simulink model "integrator_test"  (R2021b)
settings: Solver=FixedStepAuto  StartTime=0.0  StopTime=30e-4  FixedStep=4e-9  RelTol=1e-3
values from neighbouring files (symbols this model uses):
  force_func = @(x) p.alpha * x.^3 - p.beta * x    [hilsim_playground.m]
undefined symbols (not defined in the file or in its folder): hw, m, p, renorm_x
settings Model: Creator=berndorfer  LastModifiedBy=berndorfer

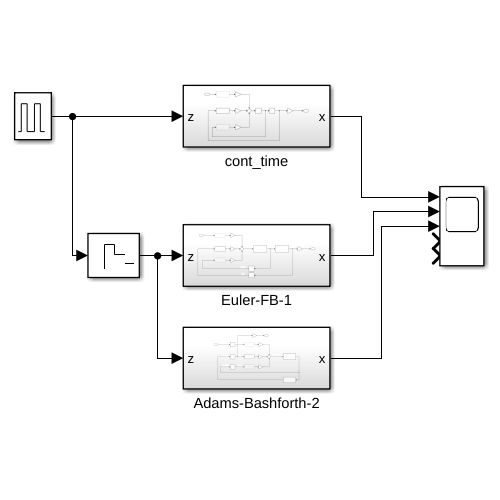
[thumbnail: Simulink's stored preview of the top-level diagram]
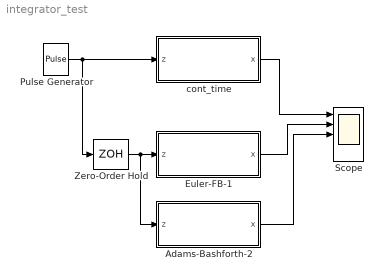
== system integrator_test ==
  Adams-Bashforth-2 : Subsystem
  Euler-FB-1 : Subsystem
  Pulse Generator : DiscretePulseGenerator  PulseType=Time based  Amplitude=-1  Period=2e-3  PulseWidth=4  PhaseDelay=0.05e-3
  Scope : Scope  NumInputPorts=5
  Zero-Order Hold : ZeroOrderHold  SampleTime=hw.t_s * hw.oversample
  cont_time : Subsystem
  wires:
  Pulse Generator/1 -> Zero-Order Hold/1, cont_time/1(z)
  cont_time/1(x) -> Scope/1
  Euler-FB-1/1(x) -> Scope/2
  Adams-Bashforth-2/1(x) -> Scope/3
  Zero-Order Hold/1 -> Adams-Bashforth-2/1(z), Euler-FB-1/1(z)

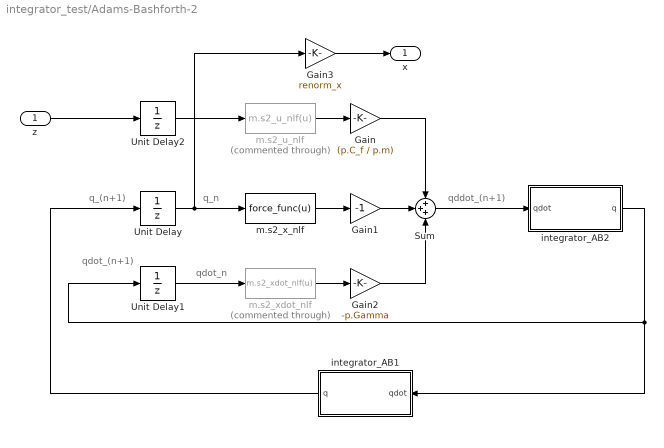
== system integrator_test/Adams-Bashforth-2 ==
  note: q_n
  note: qddot_(n+1)
  note: qdot_(n+1)
  note: qdot_n
  note: q_(n+1)
  z : Inport
  Gain : Gain  Gain=(p.C_f / p.m)
  Gain1 : Gain  Gain=-1
  Gain2 : Gain  Gain=-p.Gamma
  Gain3 : Gain  Gain=renorm_x
  Sum : Sum  Inputs=+++
  Unit Delay : UnitDelay  SampleTime=hw.t_s * hw.oversample  HasFrameUpgradeWarning=on
  Unit Delay1 : UnitDelay  SampleTime=hw.t_s * hw.oversample  HasFrameUpgradeWarning=on
  Unit Delay2 : UnitDelay  SampleTime=hw.t_s * hw.oversample  HasFrameUpgradeWarning=on
  integrator_AB1 : Subsystem
  integrator_AB2 : Subsystem
  m.s2_u_nlf : MATLABFcn  Commented=through  MATLABFcn=m.s2_u_nlf(u)  OutputDimensions=1
  m.s2_x_nlf : MATLABFcn  MATLABFcn=force_func(u)  OutputDimensions=1
  m.s2_xdot_nlf : MATLABFcn  Commented=through  MATLABFcn=m.s2_xdot_nlf(u)  OutputDimensions=1
  x : Outport
  wires:
  Gain1/1 -> Sum/2
  z/1 -> Unit Delay2/1
  Gain/1 -> Sum/1
  m.s2_x_nlf/1 -> Gain1/1
  Unit Delay/1 -> Gain3/1, m.s2_x_nlf/1
  m.s2_xdot_nlf/1 -> Gain2/1
  Gain2/1 -> Sum/3
  m.s2_u_nlf/1 -> Gain/1
  Gain3/1 -> x/1
  Unit Delay2/1 -> m.s2_u_nlf/1
  Unit Delay1/1 -> m.s2_xdot_nlf/1
  integrator_AB2/1(q) -> integrator_AB1/1(qdot), Unit Delay1/1
  integrator_AB1/1(q) -> Unit Delay/1
  Sum/1 -> integrator_AB2/1(qdot)

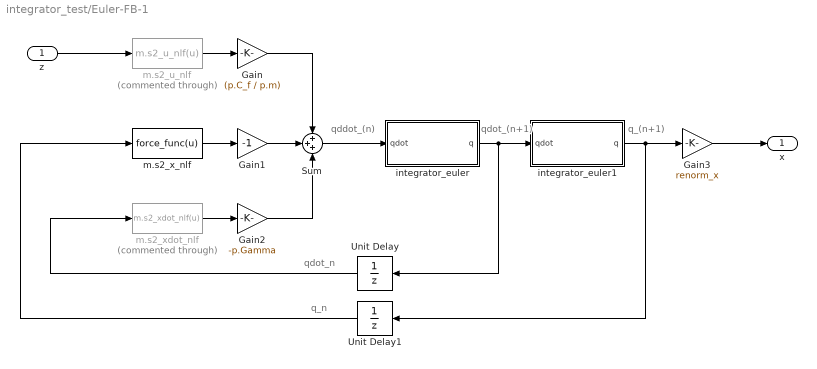
== system integrator_test/Euler-FB-1 ==
  note: qdot_n
  note: qdot_(n+1)
  note: q_(n+1)
  note: q_n
  note: qddot_(n)
  z : Inport
  Gain : Gain  Gain=(p.C_f / p.m)
  Gain1 : Gain  Gain=-1
  Gain2 : Gain  Gain=-p.Gamma
  Gain3 : Gain  Gain=renorm_x
  Sum : Sum  Inputs=+++
  Unit Delay : UnitDelay  SampleTime=hw.t_s * hw.oversample  HasFrameUpgradeWarning=on
  Unit Delay1 : UnitDelay  SampleTime=hw.t_s * hw.oversample  HasFrameUpgradeWarning=on
  integrator_euler : Subsystem
  integrator_euler1 : Subsystem
  m.s2_u_nlf : MATLABFcn  Commented=through  MATLABFcn=m.s2_u_nlf(u)  OutputDimensions=1
  m.s2_x_nlf : MATLABFcn  MATLABFcn=force_func(u)  OutputDimensions=1
  m.s2_xdot_nlf : MATLABFcn  Commented=through  MATLABFcn=m.s2_xdot_nlf(u)  OutputDimensions=1
  x : Outport
  wires:
  Gain1/1 -> Sum/2
  Gain/1 -> Sum/1
  m.s2_x_nlf/1 -> Gain1/1
  Sum/1 -> integrator_euler/1(qdot)
  m.s2_xdot_nlf/1 -> Gain2/1
  Gain2/1 -> Sum/3
  m.s2_u_nlf/1 -> Gain/1
  Gain3/1 -> x/1
  z/1 -> m.s2_u_nlf/1
  Unit Delay/1 -> m.s2_xdot_nlf/1
  Unit Delay1/1 -> m.s2_x_nlf/1
  integrator_euler1/1(q) -> Unit Delay1/1, Gain3/1
  integrator_euler/1(q) -> Unit Delay/1, integrator_euler1/1(qdot)

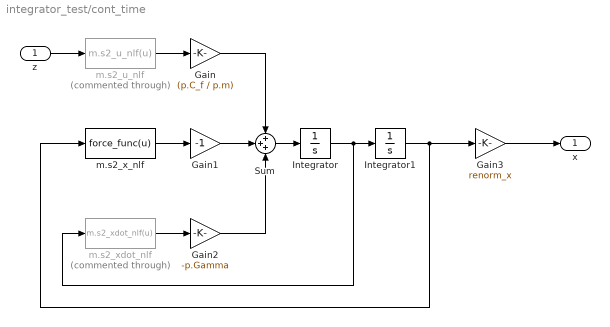
== system integrator_test/cont_time ==
  z : Inport
  Gain : Gain  Gain=(p.C_f / p.m)
  Gain1 : Gain  Gain=-1
  Gain2 : Gain  Gain=-p.Gamma
  Gain3 : Gain  Gain=renorm_x
  Integrator : Integrator
  Integrator1 : Integrator
  Sum : Sum  Inputs=+++
  m.s2_u_nlf : MATLABFcn  Commented=through  MATLABFcn=m.s2_u_nlf(u)  OutputDimensions=1
  m.s2_x_nlf : MATLABFcn  MATLABFcn=force_func(u)  OutputDimensions=1
  m.s2_xdot_nlf : MATLABFcn  Commented=through  MATLABFcn=m.s2_xdot_nlf(u)  OutputDimensions=1
  x : Outport
  wires:
  Gain1/1 -> Sum/2
  z/1 -> m.s2_u_nlf/1
  Integrator/1 -> m.s2_xdot_nlf/1, Integrator1/1
  Gain/1 -> Sum/1
  m.s2_x_nlf/1 -> Gain1/1
  Sum/1 -> Integrator/1
  Integrator1/1 -> Gain3/1, m.s2_x_nlf/1
  m.s2_xdot_nlf/1 -> Gain2/1
  Gain2/1 -> Sum/3
  m.s2_u_nlf/1 -> Gain/1
  Gain3/1 -> x/1

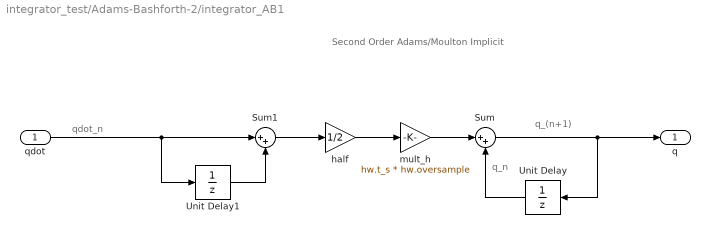
== system integrator_test/Adams-Bashforth-2/integrator_AB1 ==
  note: Second Order Adams/Moulton Implicit
  note: qdot_n
  note: q_n
  note: q_(n+1)
  qdot : Inport
  Sum : Sum  Inputs=|++
  Sum1 : Sum  Inputs=|++
  Unit Delay : UnitDelay  SampleTime=hw.t_s * hw.oversample  HasFrameUpgradeWarning=on
  Unit Delay1 : UnitDelay  SampleTime=hw.t_s * hw.oversample  HasFrameUpgradeWarning=on
  half : Gain  Gain=1/2
  mult_h : Gain  Gain=hw.t_s * hw.oversample
  q : Outport
  wires:
  mult_h/1 -> Sum/1
  Sum/1 -> Unit Delay/1, q/1
  Unit Delay/1 -> Sum/2
  qdot/1 -> Unit Delay1/1, Sum1/1
  Sum1/1 -> half/1
  Unit Delay1/1 -> Sum1/2
  half/1 -> mult_h/1

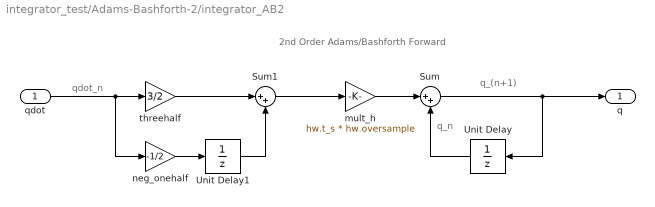
== system integrator_test/Adams-Bashforth-2/integrator_AB2 ==
  note: 2nd Order Adams/Bashforth Forward
  note: qdot_n
  note: q_n
  note: q_(n+1)
  qdot : Inport
  Sum : Sum  Inputs=|++
  Sum1 : Sum  Inputs=|++
  Unit Delay : UnitDelay  SampleTime=hw.t_s * hw.oversample  HasFrameUpgradeWarning=on
  Unit Delay1 : UnitDelay  SampleTime=hw.t_s * hw.oversample  HasFrameUpgradeWarning=on
  mult_h : Gain  Gain=hw.t_s * hw.oversample
  neg_onehalf : Gain  Gain=-1/2
  threehalf : Gain  Gain=3/2
  q : Outport
  wires:
  mult_h/1 -> Sum/1
  Sum/1 -> Unit Delay/1, q/1
  Unit Delay/1 -> Sum/2
  threehalf/1 -> Sum1/1
  neg_onehalf/1 -> Unit Delay1/1
  Sum1/1 -> mult_h/1
  qdot/1 -> neg_onehalf/1, threehalf/1
  Unit Delay1/1 -> Sum1/2

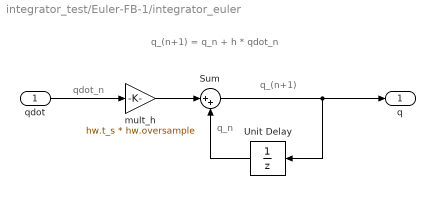
== system integrator_test/Euler-FB-1/integrator_euler ==
  note: qdot_n
  note: q_n
  note: q_(n+1)
  note: q_(n+1) = q_n + h * qdot_n
  qdot : Inport
  Sum : Sum  Inputs=|++
  Unit Delay : UnitDelay  SampleTime=hw.t_s * hw.oversample  HasFrameUpgradeWarning=on
  mult_h : Gain  Gain=hw.t_s * hw.oversample
  q : Outport
  wires:
  qdot/1 -> mult_h/1
  mult_h/1 -> Sum/1
  Sum/1 -> Unit Delay/1, q/1
  Unit Delay/1 -> Sum/2

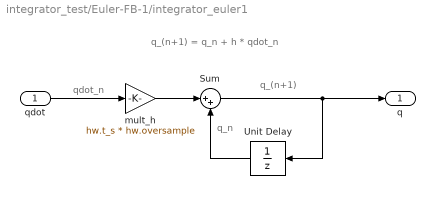
== system integrator_test/Euler-FB-1/integrator_euler1 ==
  note: qdot_n
  note: q_n
  note: q_(n+1)
  note: q_(n+1) = q_n + h * qdot_n
  qdot : Inport
  Sum : Sum  Inputs=|++
  Unit Delay : UnitDelay  SampleTime=hw.t_s * hw.oversample  HasFrameUpgradeWarning=on
  mult_h : Gain  Gain=hw.t_s * hw.oversample
  q : Outport
  wires:
  qdot/1 -> mult_h/1
  mult_h/1 -> Sum/1
  Sum/1 -> Unit Delay/1, q/1
  Unit Delay/1 -> Sum/2
